simulink model "MANDO_s4"  (R2015a)
settings: Solver=ode4  SolverMode=SingleTasking  StartTime=0.0  StopTime=inf  FixedStep=ts  RelTol=1e-3
values from neighbouring files (symbols this model uses):
  ts = 5e-3    (= 0.005)    [CONTROL_SEGWAY.m]
libraries: legonxtlib x10, simulink x2
settings Model: CovSFcnEnable=off  ExtModeTrigDuration=2  Creator=jrperez  LastModifiedBy=201505200
settings DataIOCC: SignalLoggingSaveFormat=ModelDataLogs
settings OptimizationCC: ExpressionDepthLimit=2147483647  OptimizeModelRefInitCode=on  LifeSpan=1
settings DebuggingCC: UnderspecifiedInitializationDetection=Classic  MergeDetectMultiDrivingBlocksExec=none  ParameterPrecisionLossMsg=none  FcnCallInpInsideContextMsg=EnableAllAsWarning  StateNameClashWarn=warning
settings HardwareCC: ProdLargestAtomicInteger=Long  ProdLargestAtomicFloat=Float  ProdEndianess=LittleEndian  ProdHWDeviceType=ARM Compatible->ARM 7
settings RTWCC: SystemTargetFile=realtime.tlc  GenerateMakefile=off  TemplateMakefile=realtime.tmf  Description=Real-Time Toolbox  RTWVerbose=off
settings CodeAppCC: CustomSymbolStrType=$N$R$M  InternalIdentifier=Classic
settings ERTTargetCC: CombineOutputUpdateFcns=off  ExtModeTransport=1  ExtModeMexFile=ext_serial_win32_comm_no_acks_rtt_byteswap  ExtModeMexArgs=0 7 9600  InlinedParameterPlacement=Hierarchical  ERTSrcFileBannerTemplate=realtime_code_template.cgt  ERTHdrFileBannerTemplate=realtime_code_template.cgt  ERTDataSrcFileTemplate=realtime_code_template.cgt  ERTDataHdrFileTemplate=realtime_code_template.cgt  ERTCustomFileTemplate=realtime_file_process.tlc

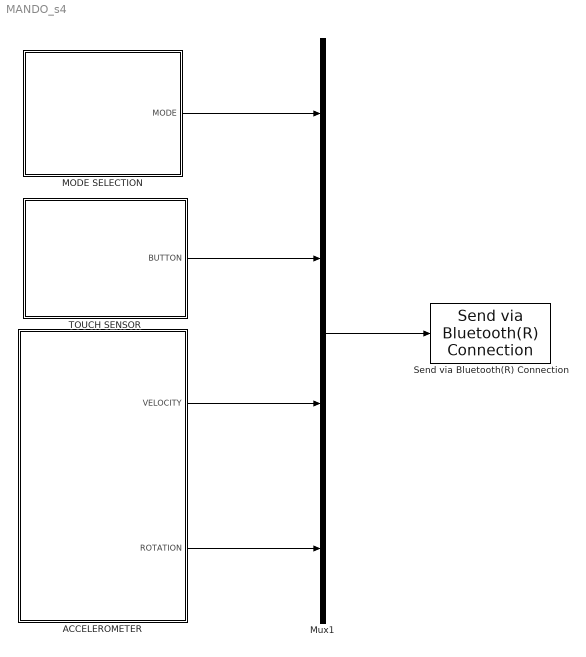
== system MANDO_s4 ==
  ACCELEROMETER : Subsystem
  MODE SELECTION : Subsystem
  Mux1 : Mux
  Send via Bluetooth(R) Connection : legonxtlib/Send via Bluetooth(R) Connection  mailbox=1  blockPlatform=LegoMindstormsNXT
  TOUCH SENSOR : Subsystem
  wires:
  Mux1/1 -> Send via Bluetooth(R) Connection/1
  TOUCH SENSOR/1(BUTTON) -> Mux1/2
  MODE SELECTION/1(MODE) -> Mux1/1
  ACCELEROMETER/1(VELOCITY) -> Mux1/3
  ACCELEROMETER/2(ROTATION) -> Mux1/4

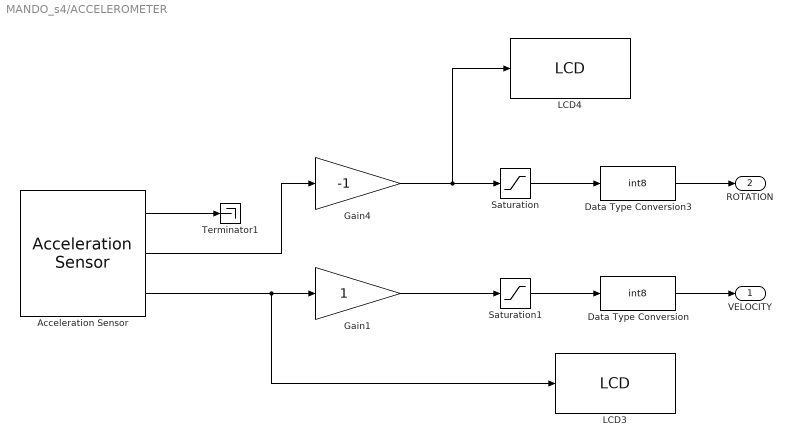
== system MANDO_s4/ACCELEROMETER ==
  Acceleration Sensor : legonxtlib/Acceleration Sensor  portNumber=4  sampleTime=ts  blockPlatform=LegoMindstormsNXT
  Data Type Conversion : DataTypeConversion  OutDataTypeStr=int8
  Data Type Conversion3 : DataTypeConversion  OutDataTypeStr=int8
  Gain1 : Gain
  Gain4 : Gain  Gain=-1
  LCD3 : legonxtlib/LCD  slcdStr=AVANCE  slcdLine=3  slcdFormat=Decimal  blockPlatform=LegoMindstormsNXT
  LCD4 : legonxtlib/LCD  slcdStr=GIRO  slcdLine=4  slcdFormat=Decimal  blockPlatform=LegoMindstormsNXT
  Saturation : Saturate  UpperLimit=100  LowerLimit=-100
  Saturation1 : Saturate  UpperLimit=100  LowerLimit=-100
  Terminator1 : Terminator
  VELOCITY : Outport
  ROTATION : Outport  Port=2
  wires:
  Data Type Conversion/1 -> VELOCITY/1
  Gain4/1 -> LCD4/1, Saturation/1
  Data Type Conversion3/1 -> ROTATION/1
  Acceleration Sensor/2 -> Gain4/1
  Acceleration Sensor/3 -> LCD3/1, Gain1/1
  Acceleration Sensor/1 -> Terminator1/1
  Saturation/1 -> Data Type Conversion3/1
  Saturation1/1 -> Data Type Conversion/1
  Gain1/1 -> Saturation1/1

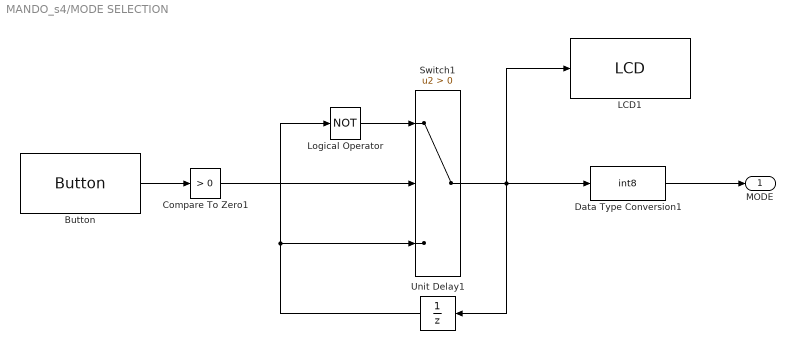
== system MANDO_s4/MODE SELECTION ==
  Button : legonxtlib/Button  buttonType=Right arrow  sampleTime=30*ts  blockPlatform=LegoMindstormsNXT
  Compare To Zero1 : simulink/Logic and Bit Operations/Compare To Zero  relop=>  OutDataTypeStr=boolean
  Data Type Conversion1 : DataTypeConversion  OutDataTypeStr=int8
  LCD1 : legonxtlib/LCD  slcdStr=MODO  slcdLine=1  slcdFormat=Decimal  blockPlatform=LegoMindstormsNXT
  Logical Operator : Logic  Operator=NOT  AllPortsSameDT=off  OutDataTypeStr=boolean
  Switch1 : Switch  Criteria=u2 > Threshold
  Unit Delay1 : UnitDelay  SampleTime=-1
  MODE : Outport  SampleTime=ts
  wires:
  Button/1 -> Compare To Zero1/1
  Switch1/1 -> Data Type Conversion1/1, LCD1/1, Unit Delay1/1
  Unit Delay1/1 -> Logical Operator/1, Switch1/3
  Compare To Zero1/1 -> Switch1/2
  Logical Operator/1 -> Switch1/1
  Data Type Conversion1/1 -> MODE/1

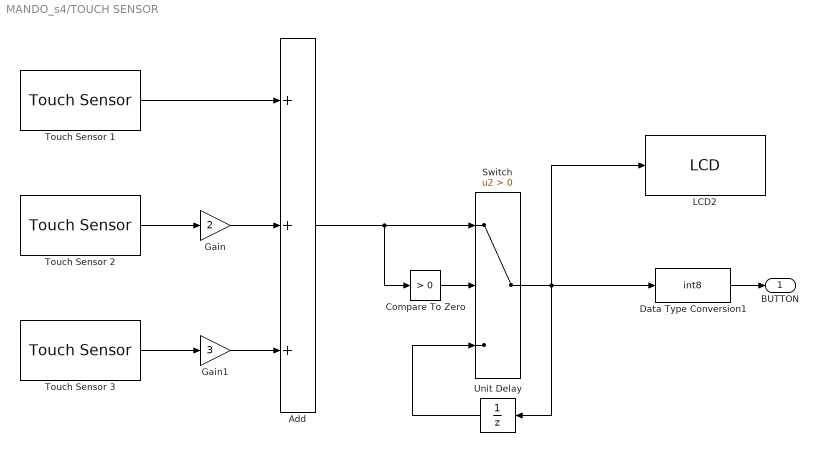
== system MANDO_s4/TOUCH SENSOR ==
  Add : Sum  Inputs=3
  Compare To Zero : simulink/Logic and Bit Operations/Compare To Zero  relop=>  OutDataTypeStr=boolean
  Data Type Conversion1 : DataTypeConversion  OutDataTypeStr=int8
  Gain : Gain  Gain=2
  Gain1 : Gain  Gain=3
  LCD2 : legonxtlib/LCD  slcdStr=PULS  slcdLine=2  slcdFormat=Decimal  blockPlatform=LegoMindstormsNXT
  Switch : Switch  Criteria=u2 > Threshold
  Touch Sensor 1 : legonxtlib/Touch Sensor  portNumber=1  sampleTime=ts  blockPlatform=LegoMindstormsNXT
  Touch Sensor 2 : legonxtlib/Touch Sensor  portNumber=2  sampleTime=ts  blockPlatform=LegoMindstormsNXT
  Touch Sensor 3 : legonxtlib/Touch Sensor  portNumber=3  sampleTime=ts  blockPlatform=LegoMindstormsNXT
  Unit Delay : UnitDelay  SampleTime=-1
  BUTTON : Outport
  wires:
  Switch/1 -> LCD2/1, Data Type Conversion1/1, Unit Delay/1
  Add/1 -> Switch/1, Compare To Zero/1
  Gain/1 -> Add/2
  Gain1/1 -> Add/3
  Unit Delay/1 -> Switch/3
  Compare To Zero/1 -> Switch/2
  Touch Sensor 2/1 -> Gain/1
  Touch Sensor 3/1 -> Gain1/1
  Touch Sensor 1/1 -> Add/1
  Data Type Conversion1/1 -> BUTTON/1
